simulink model "L_21_05_12_effetti_sul_comando_schema"  (R2021b)
settings: Solver=VariableStepAuto  StartTime=0.0  StopTime=10.0  RelTol=1e-3
values from neighbouring files (symbols this model uses):
  Kr = 1    [L_11_05_21_reti_anticipatrici.m]    (also in L_11_05_21_reti_anticipatrici_2.m; L_12_05_21_Esercizio_progetto_di_un_controllore.m; L_12_05_21_effetti_sul_comando.m; L_12_05_21_reti_integro-derivative.m)
libraries: cstblocks x2
settings Model: Creator=armandofornasier  LastModifiedBy=francescafornasier

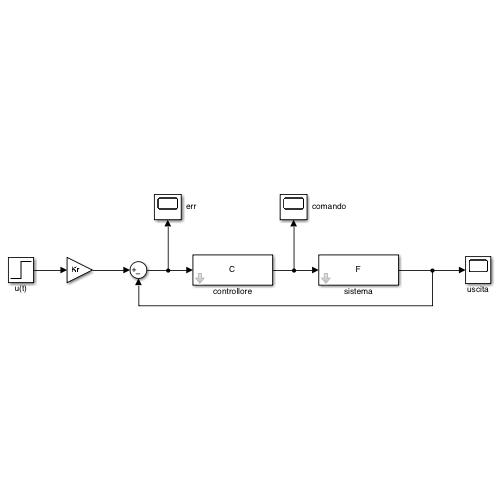
[thumbnail: Simulink's stored preview of the top-level diagram]
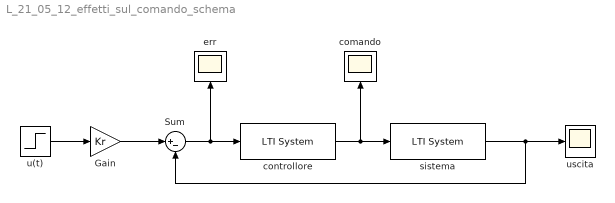
== system L_21_05_12_effetti_sul_comando_schema ==
  Gain : Gain  Gain=Kr
  Sum : Sum  Inputs=|+-
  comando : Scope
  controllore : cstblocks/LTI System  sys=C  IC=[]
  err : Scope
  sistema : cstblocks/LTI System  sys=F  IC=[]
  u(t) : Step  Time=0  SampleTime=0
  uscita : Scope
  wires:
  u(t)/1 -> Gain/1
  Gain/1 -> Sum/1
  Sum/1 -> err/1, controllore/1
  controllore/1 -> comando/1, sistema/1
  sistema/1 -> uscita/1, Sum/2
